simulink model "goodwin"  (R2021a)
settings: Solver=VariableStepAuto  StartTime=0.0  StopTime=25  RelTol=1e-6
undefined symbols (not defined in the file): A, B, C, dencl, dens, E1, G, J, K, ki, L, numcl, nums, P
libraries: simulink x1
settings Model: Creator=amnlima  LastModifiedBy=dbnun
settings SolverCC: AlgebraicLoopSolver=TrustRegion
settings DataIOCC: ReturnWorkspaceOutputs=off
settings DebuggingCC: SFMachineParentedDataDiag=warning  ArithmeticOperatorsInVariantConditions=warning
settings SFSimCC: SimUseLocalCustomCode=off  CustomCodeUndefinedFunction=UseInterfaceOnly
settings RTWCC: RTWUseLocalCustomCode=off

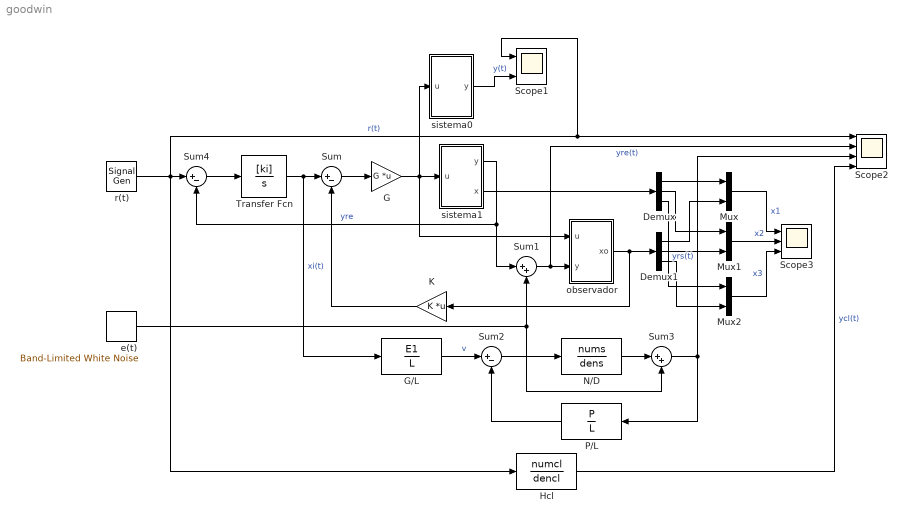
== system goodwin ==
  Demux : Demux  Outputs=3
  Demux1 : Demux  Outputs=3
  G : Gain  Gain=G  Multiplication=Matrix(K*u)
  G/L : TransferFcn  Numerator=E1  Denominator=L
  Hcl : TransferFcn  Numerator=numcl  Denominator=dencl
  K : Gain  Gain=K  Multiplication=Matrix(K*u)
  Mux : Mux  Inputs=2
  Mux1 : Mux  Inputs=2
  Mux2 : Mux  Inputs=2
  N/D : TransferFcn  Numerator=nums  Denominator=dens
  P/L : TransferFcn  Numerator=P  Denominator=L
  Scope1 : Scope  NumInputPorts=2
  Scope2 : Scope  NumInputPorts=4
  Scope3 : Scope  NumInputPorts=3
  Sum : Sum  Inputs=|+-
  Sum1 : Sum  Inputs=|++
  Sum2 : Sum  Inputs=|+-
  Sum3 : Sum  Inputs=|++
  Sum4 : Sum  Inputs=|+-
  Transfer Fcn : TransferFcn  Numerator=[ki]  Denominator=[1 0]
  e(t) : simulink/Sources/Band-Limited White Noise  Cov=[0.0]  Ts=0.1  seed=[23341]
  observador : Subsystem
  r(t) : SignalGenerator  WaveForm=square  Amplitude=-1  Frequency=0.05
  sistema0 : Subsystem
  sistema1 : Subsystem
  wires:
  sistema1/1(y) -> Sum4/2, Sum1/1  "yre"
  observador/1(xo) -> Demux1/1, K/1
  G/1 -> observador/1(u), sistema0/1(u), sistema1/1(u)
  K/1 -> Sum/2
  Transfer Fcn/1 -> G/L/1, Sum/1  "xi(t)"
  r(t)/1 -> Scope1/1, Scope2/1, Hcl/1, Sum4/1  "r(t)"
  sistema1/2(x) -> Demux/1
  Demux/1 -> Mux/1
  Demux1/1 -> Mux/2
  Demux/2 -> Mux1/1
  Demux1/2 -> Mux1/2
  Demux/3 -> Mux2/1
  Demux1/3 -> Mux2/2
  Mux/1 -> Scope3/1  "x1"
  Mux1/1 -> Scope3/2  "x2"
  Mux2/1 -> Scope3/3  "x3"
  sistema0/1(y) -> Scope1/2  "y(t)"
  Sum1/1 -> Scope2/2, observador/2(y)  "yre(t)"
  e(t)/1 -> Sum1/2, Sum3/2
  Sum2/1 -> N/D/1
  G/L/1 -> Sum2/1  "v"
  P/L/1 -> Sum2/2
  N/D/1 -> Sum3/1
  Sum3/1 -> Scope2/3, P/L/1  "yrs(t)"
  Hcl/1 -> Scope2/4  "ycl(t)"
  Sum4/1 -> Transfer Fcn/1
  Sum/1 -> G/1

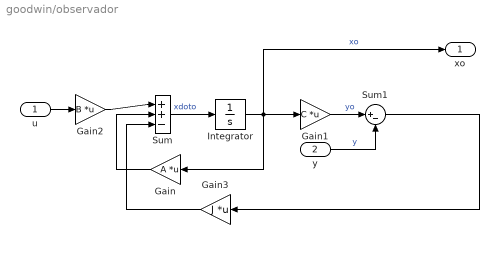
== system goodwin/observador ==
  u : Inport
  y : Inport  Port=2
  Gain : Gain  Gain=A  Multiplication=Matrix(K*u)
  Gain1 : Gain  Gain=C  Multiplication=Matrix(K*u)
  Gain2 : Gain  Gain=B  Multiplication=Matrix(K*u)
  Gain3 : Gain  Gain=J  Multiplication=Matrix(K*u)
  Integrator : Integrator  InitialCondition=[0;0;0]
  Sum : Sum  Inputs=|++-
  Sum1 : Sum  Inputs=|+-
  xo : Outport  VectorParamsAs1DForOutWhenUnconnected=off
  wires:
  u/1 -> Gain2/1
  Gain1/1 -> Sum1/1  "yo"
  Sum/1 -> Integrator/1  "xdoto"
  Gain2/1 -> Sum/1
  Gain/1 -> Sum/2
  Integrator/1 -> Gain1/1, xo/1, Gain/1  "xo"
  y/1 -> Sum1/2  "y"
  Sum1/1 -> Gain3/1
  Gain3/1 -> Sum/3

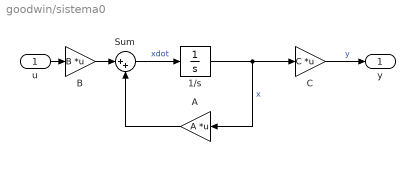
== system goodwin/sistema0 ==
  u : Inport
  1/s : Integrator  InitialCondition=[0;0;0]
  A : Gain  Gain=A  Multiplication=Matrix(K*u)
  B : Gain  Gain=B  Multiplication=Matrix(K*u)
  C : Gain  Gain=C  Multiplication=Matrix(K*u)
  Sum : Sum  Inputs=|++
  y : Outport  VectorParamsAs1DForOutWhenUnconnected=off
  wires:
  u/1 -> B/1
  C/1 -> y/1  "y"
  Sum/1 -> 1/s/1  "xdot"
  B/1 -> Sum/1
  A/1 -> Sum/2
  1/s/1 -> C/1, A/1  "x"

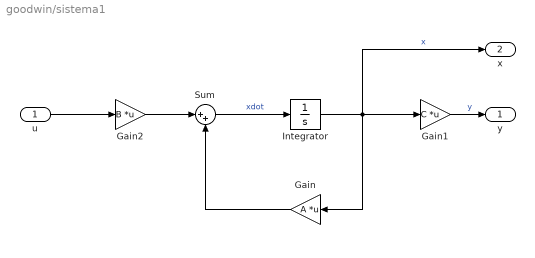
== system goodwin/sistema1 ==
  u : Inport
  Gain : Gain  Gain=A  Multiplication=Matrix(K*u)
  Gain1 : Gain  Gain=C  Multiplication=Matrix(K*u)
  Gain2 : Gain  Gain=B  Multiplication=Matrix(K*u)
  Integrator : Integrator  InitialCondition=[0;0;0]
  Sum : Sum  Inputs=|++
  y : Outport  VectorParamsAs1DForOutWhenUnconnected=off
  x : Outport  Port=2  VectorParamsAs1DForOutWhenUnconnected=off
  wires:
  u/1 -> Gain2/1
  Gain1/1 -> y/1  "y"
  Sum/1 -> Integrator/1  "xdot"
  Gain2/1 -> Sum/1
  Gain/1 -> Sum/2
  Integrator/1 -> x/1, Gain1/1, Gain/1  "x"
